simulink model "JKFF"  (R2025b)
settings: Solver=VariableStepAuto  StartTime=0.0  StopTime=Inf  RelTol=1e-3
settings Model: Creator=Soochan Kim  LastModifiedBy=Soochan Kim

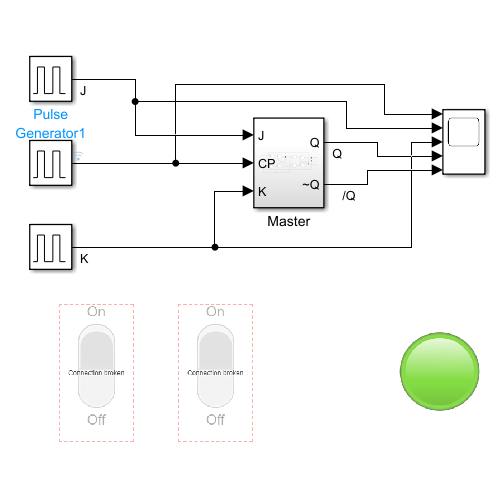
[thumbnail: Simulink's stored preview of the top-level diagram]
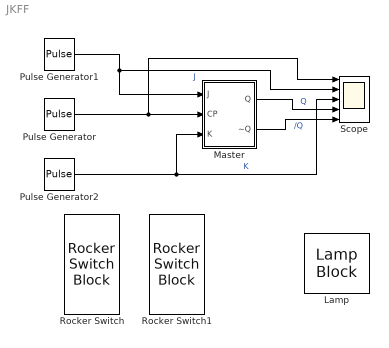
== system JKFF ==
  Lamp : LampBlock  LabelPosition=Hide  DefaultColor=[192.0, 192.0, 192.0]
  Master : Subsystem
  Pulse Generator : DiscretePulseGenerator  PulseType=Time based  Period=1  PulseWidth=50
  Pulse Generator1 : DiscretePulseGenerator  PulseType=Time based  PulseWidth=50
  Pulse Generator2 : DiscretePulseGenerator  PulseType=Time based  Period=4  PulseWidth=50
  Rocker Switch : RockerSwitchBlock
  Rocker Switch1 : RockerSwitchBlock
  Scope : Scope  NumInputPorts=5
      settings: ActiveDisplayYMinimum=-0.12499999999999997  ActiveDisplayYMaximum=1.125
  wires:
  Master/1(Q) -> Scope/4  "Q"
  Pulse Generator1/1 -> Master/1(J), Scope/2  "J"
  Pulse Generator/1 -> Scope/1, Master/2(CP)
  Pulse Generator2/1 -> Master/3(K), Scope/3  "K"
  Master/2(~Q) -> Scope/5  "/Q"

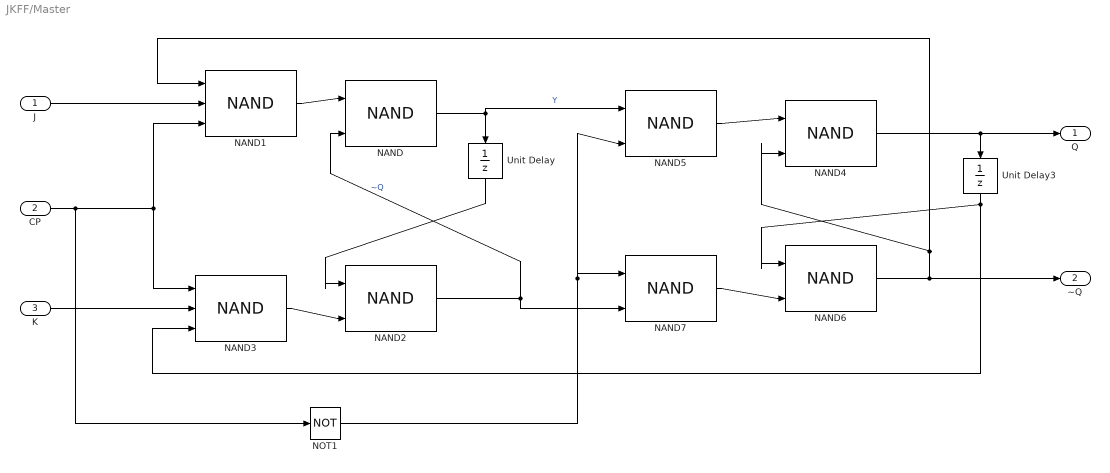
== system JKFF/Master ==
  J : Inport
  CP : Inport  Port=2
  K : Inport  Port=3
  NAND{,2,4..7} (6 alike) : Logic  Operator=NAND  IconShape=distinctive  AllPortsSameDT=off  OutDataTypeStr=boolean
  NAND1 : Logic  Operator=NAND  Inputs=3  IconShape=distinctive  AllPortsSameDT=off  OutDataTypeStr=boolean
  NAND3 : Logic  Operator=NAND  Inputs=3  IconShape=distinctive  AllPortsSameDT=off  OutDataTypeStr=boolean
  NOT1 : Logic  Operator=NOT  IconShape=distinctive  AllPortsSameDT=off  OutDataTypeStr=boolean
  Unit Delay : UnitDelay  SampleTime=0.001  HasFrameUpgradeWarning=on
  Unit Delay3 : UnitDelay  SampleTime=-1  HasFrameUpgradeWarning=on
  Q : Outport
  ~Q : Outport  Port=2
  wires:
  NAND/1 -> Unit Delay/1, NAND5/1  "Y"
  NAND2/1 -> NAND/2, NAND7/2  "~Q"
  Unit Delay/1 -> NAND2/1
  K/1 -> NAND3/2
  NAND1/1 -> NAND/1
  NAND3/1 -> NAND2/2
  J/1 -> NAND1/2
  NAND6/1 -> ~Q/1, NAND1/1, NAND4/2
  Unit Delay3/1 -> NAND3/3, NAND6/1
  NAND5/1 -> NAND4/1
  NAND7/1 -> NAND6/2
  NAND4/1 -> Q/1, Unit Delay3/1
  CP/1 -> NAND1/3, NAND3/1, NOT1/1
  NOT1/1 -> NAND5/2, NAND7/1
